simulink model "FSM_parking_gate_v2"  (R2024a)
settings: Solver=FixedStepAuto  StartTime=0.0  StopTime=100  FixedStep=0.2  RelTol=1e-3
settings Model: PacingRate=2  Creator=ArriGE66  LastModifiedBy=Bocchio
settings ModelReferenceCC: EnableRefExpFcnMdlSchedulingChecks=on
settings RTWCC: GPUComputeCapability=3.5

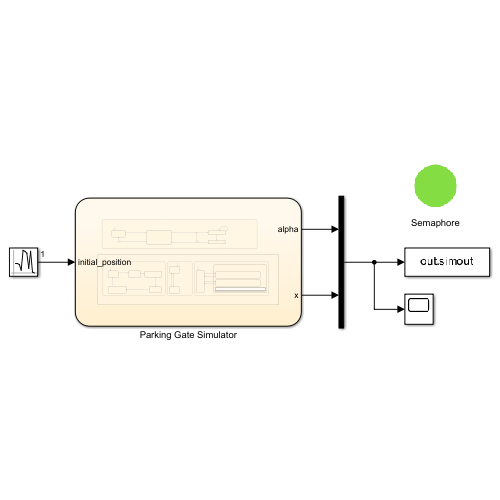
[thumbnail: Simulink's stored preview of the top-level diagram]
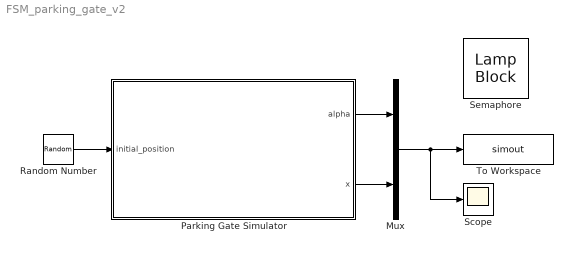
== system FSM_parking_gate_v2 ==
  Mux : Mux  Inputs=2
  Parking Gate Simulator : Stateflow chart  TreatAsAtomicUnit=on
  Random Number : RandomNumber  Mean=-15  Variance=5  SampleTime=0.2
  Scope : Scope
  Semaphore : LampBlock  LabelPosition=Hide  Icon=Circle
  To Workspace : ToWorkspace  VariableName=simout  SampleTime=-1
  wires:
  Random Number/1 -> Parking Gate Simulator/1(initial_position)
  Parking Gate Simulator/1(alpha) -> Mux/1
  Parking Gate Simulator/2(x) -> Mux/2
  Mux/1 -> To Workspace/1, Scope/1

== stateflow chart FSM_parking_gate_v2/Parking Gate Simulator ==
  state Car [parallel]
    settings: executionOrder=1
    state Paying
      entry: send(PayTicket);
    state Driving
      during:
      v = min(abs(x), 30/3.6)  + 10e-2;
      x = min(x + v*dt, checkpoint);
    state Spawning
      entry: x = initial_position;
    state Waiting
    (default) -> Spawning
    Paying -> Paying [order 2] : [after(2, sec)]
    Driving -> (junction 169) [order 1] : [x == checkpoint]
    (junction 169) -> Paying [order 1] : [~gate_up]
    Spawning -> Driving : {checkpoint = gate_x;}
    (junction 169) -> (junction 171) [order 2]
    Paying -> Waiting [order 1] : [auth]
    (junction 130) -> Spawning : after(2, sec)
    Driving -> (junction 130) [order 2] : [x > gate_x && ~gate_up]
    (junction 171) -> Driving : [gate_up]{checkpoint = +inf;}
    Waiting -> (junction 171)
  state Parking gate logic [group]
    state Controller [parallel]
      settings: executionOrder=1
      state Idling
        entry: auth = false
      state Authorizing
        entry: auth = true;
      state GateClosing
        entry: send(LowerGate);
      state GateOpening
        entry: send(RaiseGate)
      state WaitingClearance
      (default) -> Parking.Controller.Idling
      Parking.Controller.Idling -> Authorizing : PayTicket
      GateClosing -> Parking.Controller.Idling : [~gate_up]
      Authorizing -> GateOpening
      WaitingClearance -> GateClosing : [in(PhotoCell.Free)]
      GateOpening -> WaitingClearance : [gate_up]
    state PhotoCell [parallel]
      settings: executionOrder=2
      state Free
      state Occupied
      (default) -> Free
      Occupied -> Free : [
          |   x<=(gate_x - 50e-2) || ...
          |   x>=(gate_x + car_length)
          | ]
      Free -> Occupied : [
          |   x>(gate_x - 50e-2) && ...
          |   x<(gate_x + car_length)
          | ]
    state Gate [parallel]
      settings: executionOrder=3
      state Moving
        state Raising
          entry: [time, alphas] = computeTrapezoidalProfile(alpha, 90, max_omega, max_omega_dot);
          during: alpha = interp1(time, alphas, elapsed(sec), 'nearest', 'extrap');
          exit: gate_up = true;
        state Lowering
          entry: [time, alphas] = computeTrapezoidalProfile(alpha, 0, max_omega, max_omega_dot);
          during: alpha = interp1(time, alphas, elapsed(sec), 'nearest', 'extrap');
          exit: gate_up = false;
      state Idling
      (default) -> Parking.Gate.Idling : {
          |   gate_up = false;
          |   alpha = 0;
          | }
      Parking.Gate.Idling -> Raising [order 1] : RaiseGate
      Raising -> Parking.Gate.Idling : [alpha == 90]
      Parking.Gate.Idling -> Lowering [order 2] : LowerGate
      Lowering -> Parking.Gate.Idling : [alpha == 0]
  data: pos_current function_input; pos_target function_input; max_vel function_input; max_acc function_input; t_vec function_output; x_vec function_output; initial_position input double; dt constant double =0.2; max_omega_dot constant double =1; max_omega constant double =4; v local double; car_length constant double =3; alpha output double =0; x output double; checkpoint local double; gate_x constant double =0; gate_up local boolean; auth local boolean; time local; alphas local
  events: RaiseGate local FUNCTION_CALL_EVENT; LowerGate local FUNCTION_CALL_EVENT; PayTicket local FUNCTION_CALL_EVENT
  function [t_vec, x_vec] = computeTrapezoidalProfile(pos_current, pos_target, max_vel, max_acc):
    | function [t_vec, x_vec] = computeTrapezoidalProfile(pos_current, pos_target, max_vel, max_acc)
    | % COMPUTE_TRAPEZOIDAL_PROFILE Generates time and angle points for a trapezoidal profile
    | % At first checks if a trapezoidal profile is feasible or is necessary to
    | % fallback to a triangular one.
    | 
    | delta_pos = pos_target - pos_current;
    | time_acc_phase = max_vel / max_acc;
    | delta_pos_acc_phase = 0.5 * max_acc * time_acc_phase^2;
    | 
    | if 2 * delta_pos_acc_phase < abs(delta_pos)
    |     % Trapezoidal profile
    |     t1 = time_acc_phase;
    |     t2 = (abs(delta_pos) - 2 * delta_pos_acc_phase) / max_vel;
    |     t3 = time_acc_phase;
    | else
    |     % Triangular profile
    |     max_vel = sqrt(abs(delta_pos) * max_acc);
    |     t1 = max_vel / max_acc;
    |     t2 = 0;
    |     t3 = max_vel / max_acc;
    | end
    | 
    | 
    | % Trapezoidal profile template (HP: s0 = 0, v0 = 0)
    | acc = max_acc * sign(delta_pos);
    | vel = max_vel * sign(delta_pos);
    | profile_template = @(t) ...
    |     (t <= t1) .*                             (1/2 * acc * t.^2) + ...
    |     (t > t1 & t <= (t1 + t2)) .*             (1/2 * acc * t1^2 + vel * (t - t1)) + ...
    |     (t > (t1 + t2) & t <= (t1 + t2 + t3)) .* (1/2 * acc * t1^2 + vel * t2 + vel * (t - (t2 + t1)) - 1/2 * acc * (t - (t1 + t2)).^2) + ...
    |     (t > (t1 + t2 + t3)) .*                  (1/2 * acc * t1^2 + vel * t2 + vel * t3 - 1/2 * acc * t3.^2);
    | 
    | % Profile generation
    | t_vec = linspace(0, t1 + t2 + t3, 100);
    | x_vec = profile_template(t_vec) + pos_current;
    | 
    | end
